simulink model "sim_plant"  (R2023a)
settings: configuration reference "config" (kept outside this file)
model workspace (MATLAB code in the model file):
  | cmdLim = Simulink.Parameter;
  | cmdLim.Value = 15;
  | cmdLim.Description = 'Limit for controlling the maximum surface command angle.';
  | cmdLim.Min = 0;
  | cmdLim.Max = 90;
  | cmdLim.DocUnits = 'deg';
  | 
  | dispGain = Simulink.Parameter;
  | dispGain.Value = 0.75;
  | dispGain.Description = 'Gain applied to the displacement error.';
  | dispGain.Min = 0;
  | dispGain.Max = [];
  | dispGain.DocUnits = 'deg/sec/deg';
  | 
  | dispLim = Simulink.Parameter;
  | dispLim.Value = 30;
  | dispLim.Description = 'Limit for controlling the maximum commanded angle.';
  | dispLim.Min = 0;
  | dispLim.Max = 180;
  | dispLim.DocUnits = 'deg';
  | 
  | intGain = Simulink.Parameter;
  | intGain.Value = 0.5;
  | intGain.Description = 'Gain applied to the integral error.';
  | intGain.Min = 0;
  | intGain.Max = [];
  | intGain.DocUnits = 'deg/sec/deg/sec';
  | 
  | intLim = Simulink.Parameter;
  | intLim.Value = 5;
  | intLim.Description = 'Limit for controlling the maximum commanded angle.';
  | intLim.Min = 0;
  | intLim.Max = 90;
  | intLim.DocUnits = 'deg';
  | 
  | rateGain = Simulink.Parameter;
  | rateGain.Value = 2;
  | rateGain.Description = 'Gain applied to the rate error.';
  | rateGain.Min = 0;
  | rateGain.Max = [];
  | rateGain.DocUnits = 'deg/deg/sec';
  | 
  | rateLim = Simulink.Parameter;
  | rateLim.Value = 6;
  | rateLim.Description = 'Limit for controlling the maximum commanded angle.';
  | rateLim.Min = 0;
  | rateLim.Max = 180;
  | rateLim.DocUnits = 'deg/sec';
  | 
  | hdgGain = Simulink.Parameter;
  | hdgGain.Value = 0.015;
libraries: eeTransforms x2, servo_hub_lib x1
settings Model: RequirementInfo={} %GIDa_fe9045fd_0412_4b6e_8206_617cc20e6fde  DataDictionary=model_config.sldd  Creator=Administrator  LastModifiedBy=Administrator
settings ConfigSetRef: SourceName=config

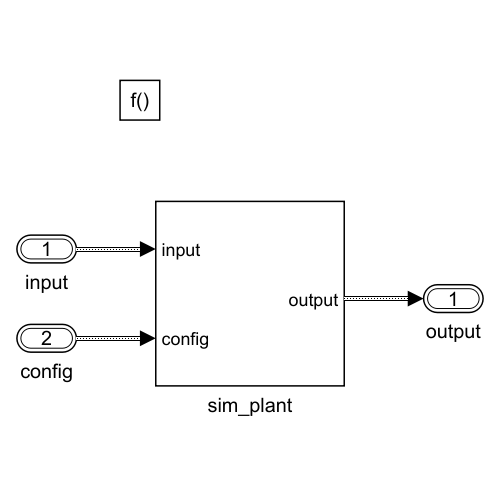
[thumbnail: Simulink's stored preview of the top-level diagram]
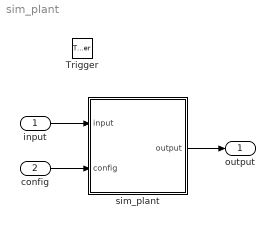
== system sim_plant ==
  input : Inport  OutDataTypeStr=Bus: SimPlantInput  BusOutputAsStruct=on
  config : Inport  Port=2  OutDataTypeStr=Bus: SimPlantConfig  BusOutputAsStruct=on
  Trigger : TriggerPort  TriggerType=function-call  VariantControl=(inherit)  PortDimensions=1
  sim_plant : Subsystem
  output : Outport  OutDataTypeStr=Bus: SimPlantOutput  BusOutputAsStruct=on
  wires:
  config/1 -> sim_plant/2(config)
  input/1 -> sim_plant/1(input)
  sim_plant/1(output) -> output/1

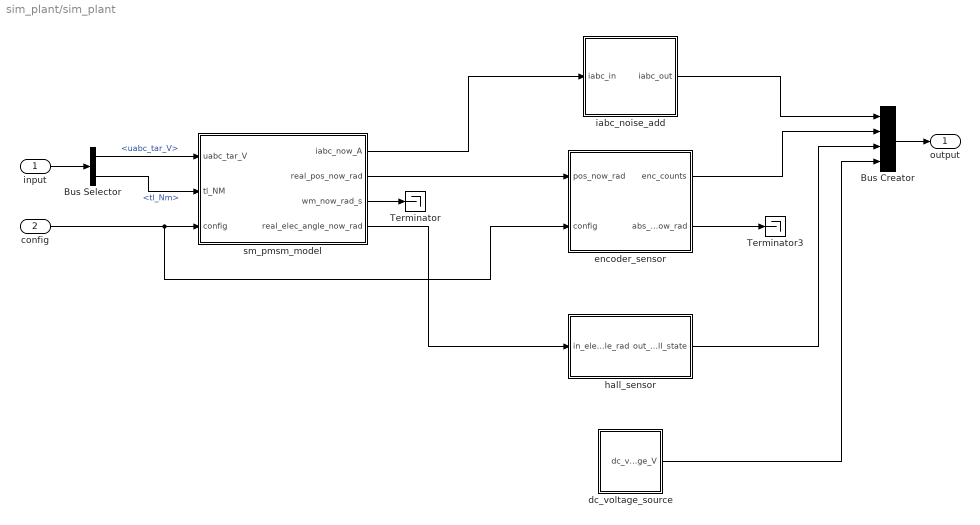
== system sim_plant/sim_plant ==
  input : Inport
  config : Inport  Port=2
  Bus Creator : BusCreator  Inputs=4  OutDataTypeStr=Bus: SimPlantOutput  NonVirtualBus=on
      settings: InheritFromInputs=off
  Bus Selector : BusSelector  OutputSignals=uabc_tar_V,tl_Nm
  Terminator : Terminator
  Terminator3 : Terminator
  dc_voltage_source : Subsystem
  encoder_sensor : Subsystem
  hall_sensor : Subsystem
  iabc_noise_add : Subsystem
  sm_pmsm_model : Subsystem
  output : Outport
  wires:
  sm_pmsm_model/2(real_pos_now_rad) -> encoder_sensor/1(pos_now_rad)
  Bus Selector/1 -> sm_pmsm_model/1(uabc_tar_V)  "<uabc_tar_V>"
  sm_pmsm_model/3(wm_now_rad_s) -> Terminator/1
  encoder_sensor/1(enc_counts) -> Bus Creator/2
  encoder_sensor/2(abs_pos_now_rad) -> Terminator3/1
  config/1 -> encoder_sensor/2(config), sm_pmsm_model/3(config)
  hall_sensor/1(out_hall_state) -> Bus Creator/3
  Bus Selector/2 -> sm_pmsm_model/2(tl_NM)  "<tl_Nm>"
  sm_pmsm_model/4(real_elec_angle_now_rad) -> hall_sensor/1(in_elec_angle_rad)
  Bus Creator/1 -> output/1
  input/1 -> Bus Selector/1
  sm_pmsm_model/1(iabc_now_A) -> iabc_noise_add/1(iabc_in)
  iabc_noise_add/1(iabc_out) -> Bus Creator/1
  dc_voltage_source/1(dc_voltage_V) -> Bus Creator/4

== system sim_plant/sim_plant/dc_voltage_source ==
  Add : Sum
  Data Type Conversion1 : DataTypeConversion  OutDataTypeStr=single  SaturateOnIntegerOverflow=off  RndMeth=Floor
  Uniform Random Number1 : UniformRandomNumber  Seed=4
  dc_bus_noise_V : Gain  Gain=0.1
  dc_voltage_base : Constant  Value=48  OutDataTypeStr=single  SampleTime=-1
  dc_voltage_V : Outport
  wires:
  dc_voltage_base/1 -> Add/1
  dc_bus_noise_V/1 -> Add/2  "noise"
  Uniform Random Number1/1 -> Data Type Conversion1/1
  Add/1 -> dc_voltage_V/1
  Data Type Conversion1/1 -> dc_bus_noise_V/1

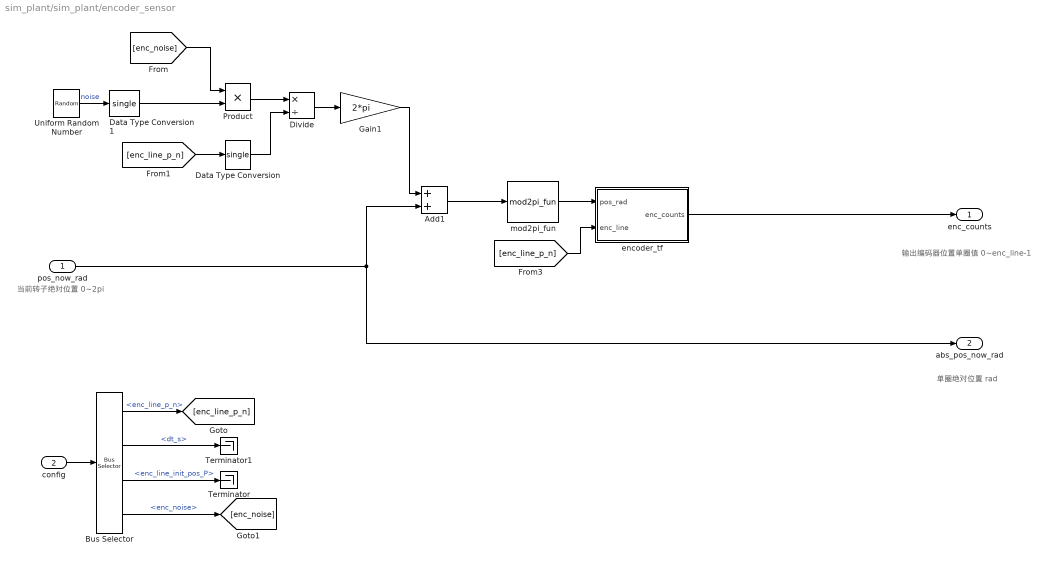
== system sim_plant/sim_plant/encoder_sensor ==
  note: 当前转子绝对位置 0~2pi
  note: 单圈绝对位置 rad
  note: 输出编码器位置单圈值 0~enc_line-1
  pos_now_rad : Inport
  config : Inport  Port=2
  Add1 : Sum
  Bus Selector : BusSelector  OutputSignals=enc_line_p_n,dt_s,enc_line_init_pos_P,enc_noise
  Data Type Conversion : DataTypeConversion  OutDataTypeStr=single  SaturateOnIntegerOverflow=off  RndMeth=Floor
  Data Type Conversion1 : DataTypeConversion  OutDataTypeStr=single  SaturateOnIntegerOverflow=off  RndMeth=Floor
  Divide : Product  Inputs=*/
  Gain1 : Gain  Gain=2*pi
  Product : Product
  Terminator : Terminator
  Terminator1 : Terminator
  Uniform Random Number : UniformRandomNumber
  encoder_tf : Subsystem
  mod2pi_fun : servo_hub_lib/fast_math/mod2pi_fun  SystemSampleTime=-1  VariantActivationTime=update diagram  Latency=0  AutoFrameSizeCalculation=off
      settings: LibrarySourceBlock=|
      | simulink/User-Defined
      | Functions/MATLAB Function
  enc_counts : Outport
  abs_pos_now_rad : Outport  Port=2
  wires:
  Data Type Conversion1/1 -> Product/2
  Uniform Random Number/1 -> Data Type Conversion1/1  "noise"
  encoder_tf/1(enc_counts) -> enc_counts/1
  Add1/1 -> mod2pi_fun/1
  mod2pi_fun/1 -> encoder_tf/1(pos_rad)
  pos_now_rad/1 -> Add1/2, abs_pos_now_rad/1
  Product/1 -> Divide/1
  [enc_line_p_n] -> Data Type Conversion/1
  Divide/1 -> Gain1/1
  config/1 -> Bus Selector/1
  Bus Selector/1 -> [enc_line_p_n]  "<enc_line_p_n>"
  Bus Selector/2 -> Terminator1/1  "<dt_s>"
  Bus Selector/3 -> Terminator/1  "<enc_line_init_pos_P>"
  Bus Selector/4 -> [enc_noise]  "<enc_noise>"
  [enc_noise] -> Product/1
  [enc_line_p_n] -> encoder_tf/2(enc_line)
  Data Type Conversion/1 -> Divide/2
  Gain1/1 -> Add1/1

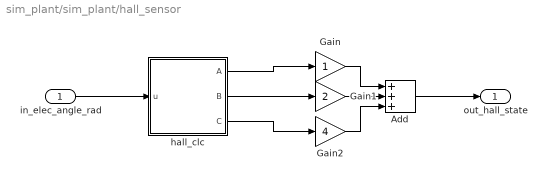
== system sim_plant/sim_plant/hall_sensor ==
  in_elec_angle_rad : Inport  OutDataTypeStr=single
  Add : Sum  Inputs=+++
  Gain : Gain  OutDataTypeStr=uint8
  Gain1 : Gain  Gain=2  OutDataTypeStr=uint8
  Gain2 : Gain  Gain=4  OutDataTypeStr=uint8
  hall_clc : MATLAB Function  TreatAsAtomicUnit=on
  out_hall_state : Outport  OutDataTypeStr=uint8
  wires:
  hall_clc/3(C) -> Gain2/1
  Add/1 -> out_hall_state/1
  hall_clc/1(A) -> Gain/1
  Gain1/1 -> Add/2
  Gain/1 -> Add/1
  in_elec_angle_rad/1 -> hall_clc/1(u)
  hall_clc/2(B) -> Gain1/1
  Gain2/1 -> Add/3

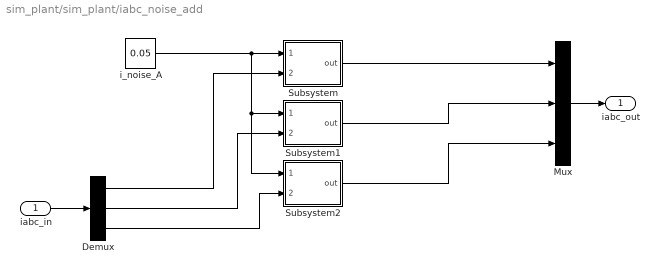
== system sim_plant/sim_plant/iabc_noise_add ==
  iabc_in : Inport
  Demux : Demux  Outputs=3
  Mux : Mux  Inputs=3
  Subsystem : Subsystem  TreatAsAtomicUnit=on
  Subsystem1 : Subsystem  TreatAsAtomicUnit=on
  Subsystem2 : Subsystem  TreatAsAtomicUnit=on
  i_noise_A : Constant  Value=0.05  OutDataTypeStr=single
  iabc_out : Outport
  wires:
  iabc_in/1 -> Demux/1
  Mux/1 -> iabc_out/1
  i_noise_A/1 -> Subsystem2/1(noise_amp), Subsystem1/1(noise_amp), Subsystem/1(noise_amp)
  Demux/1 -> Subsystem/2(source)
  Subsystem/1(out) -> Mux/1
  Subsystem1/1(out) -> Mux/2
  Subsystem2/1(out) -> Mux/3
  Demux/2 -> Subsystem1/2(source)
  Demux/3 -> Subsystem2/2(source)

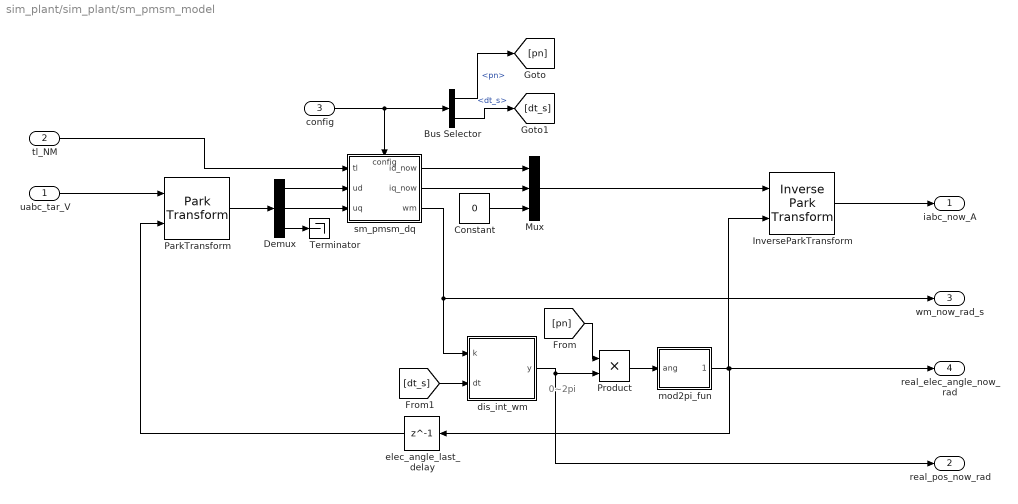
== system sim_plant/sim_plant/sm_pmsm_model ==
  note: 0~2pi
  uabc_tar_V : Inport  OutDataTypeStr=single  PortDimensions=3
  tl_NM : Inport  Port=2  OutDataTypeStr=single
  config : Inport  Port=3
  Bus Selector : BusSelector  OutputSignals=pn,dt_s
  Constant : Constant  Value=0  OutDataTypeStr=single  SampleTime=-1
  Demux : Demux  Outputs=3
  InverseParkTransform : eeTransforms/Inverse Park Transform  AxisAlignment=D-axis  PowerInvariant=off
      settings: LibrarySourceBlock=|
      | ee_sl_lib/Mathematical
      | Transforms/Inverse
      | Park Transform
  Mux : Mux  Inputs=3
  ParkTransform : eeTransforms/Park Transform  AxisAlignment=D-axis  PowerInvariant=off
      settings: LibrarySourceBlock=|
      | ee_sl_lib/Mathematical
      | Transforms/Park Transform
  Product : Product
  Terminator : Terminator
  dis_int_wm : Subsystem
  elec_angle_last_delay : Delay  DelayLength=1  StateName=elec_angle_last
  mod2pi_fun : MATLAB Function
  sm_pmsm_dq : Subsystem
      settings: PortSchema="{\"entries\":[{\"content\":{\"sides\":[{\"content\":{\"connectorIds\":[\"In1\",\"In2\",\"In3\"]},\"type\":\"ConnectorPlacement.EquallySpacedRectSide\",\"uuid\":\"d8cc84ce-9f3b-47a0-8bee-f47dde5345ac\"},{\"content\":{\"connectorIds\":[\"Out1\",\"Out2\",\"Out3\"],\"side\":\"RIGHT\"},\"type\":\"ConnectorPlacement.EquallySpacedRectSide\",\"uuid\":\"7a05c8dd-b607-4215-ae3a-55de450e01b9\"},{\"content\":{\"connectorIds\":[\"In4\"],\"side\":\"TOP\"},\"type\":\"ConnectorPlacement.EquallySpacedRectSide\",\"uuid\":\"29e5b71a-7e7a-40d5-8a8d-08d5a436dd58\"}]},\"type\":\"ConnectorPlacement.EquallySpacedConnector\",\"uuid\":\"95edc6c6-16f9-4a9f-9bec-fe8bb0215fcd\"}],\"packageUris\":[\"http://schema.mathworks.com/mf0/Connector/R2020b\"],\"version\":\"1.0\"}"
  iabc_now_A : Outport  OutDataTypeStr=single
  real_pos_now_rad : Outport  Port=2  OutDataTypeStr=single
  wm_now_rad_s : Outport  Port=3  OutDataTypeStr=single
  real_elec_angle_now_rad : Outport  Port=4  OutDataTypeStr=single
  wires:
  sm_pmsm_dq/2(iq_now) -> Mux/2
  InverseParkTransform/1 -> iabc_now_A/1
  Demux/3 -> Terminator/1
  sm_pmsm_dq/1(id_now) -> Mux/1
  sm_pmsm_dq/3(wm) -> dis_int_wm/1(k), wm_now_rad_s/1
  Constant/1 -> Mux/3
  Demux/2 -> sm_pmsm_dq/3(uq)
  Demux/1 -> sm_pmsm_dq/2(ud)
  dis_int_wm/1(y) -> real_pos_now_rad/1, Product/2
  tl_NM/1 -> sm_pmsm_dq/1(tl)
  ParkTransform/1 -> Demux/1
  Mux/1 -> InverseParkTransform/1
  uabc_tar_V/1 -> ParkTransform/1
  Product/1 -> mod2pi_fun/1(ang)
  mod2pi_fun/1(n_ang) -> InverseParkTransform/2, elec_angle_last_delay/1, real_elec_angle_now_rad/1
  elec_angle_last_delay/1 -> ParkTransform/2
  config/1 -> Bus Selector/1, sm_pmsm_dq/4(config)
  Bus Selector/1 -> [pn]  "<pn>"
  [pn] -> Product/1
  Bus Selector/2 -> [dt_s]  "<dt_s>"
  [dt_s] -> dis_int_wm/2(dt)

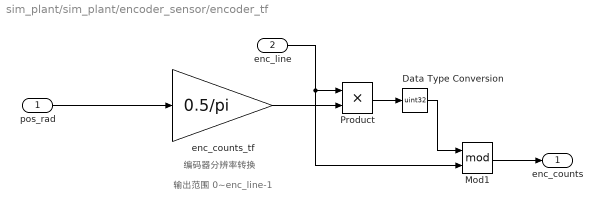
== system sim_plant/sim_plant/encoder_sensor/encoder_tf ==
  note: 输出范围 0~enc_line-1
  note: 编码器分辨率转换
  pos_rad : Inport  OutDataTypeStr=single
  enc_line : Inport  Port=2
  Data Type Conversion : DataTypeConversion  OutDataTypeStr=uint32  SaturateOnIntegerOverflow=off  RndMeth=Floor
  Mod1 : Math  Operator=mod
  Product : Product
  enc_counts_tf : Gain  Gain=0.5/pi
  enc_counts : Outport
  wires:
  enc_counts_tf/1 -> Product/2
  pos_rad/1 -> enc_counts_tf/1
  enc_line/1 -> Mod1/2, Product/1
  Mod1/1 -> enc_counts/1
  Product/1 -> Data Type Conversion/1
  Data Type Conversion/1 -> Mod1/1

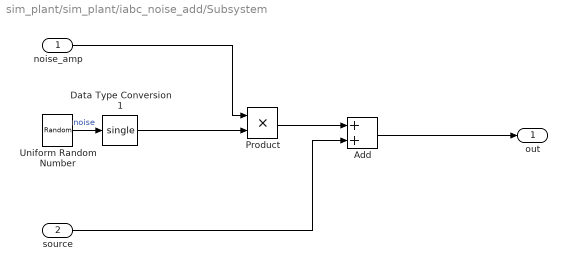
== system sim_plant/sim_plant/iabc_noise_add/Subsystem ==
  noise_amp : Inport
  source : Inport  Port=2
  Add : Sum
  Data Type Conversion1 : DataTypeConversion  OutDataTypeStr=single  SaturateOnIntegerOverflow=off  RndMeth=Floor
  Product : Product
  Uniform Random Number : UniformRandomNumber  Seed=1
  out : Outport
  wires:
  Product/1 -> Add/1
  Uniform Random Number/1 -> Data Type Conversion1/1  "noise"
  Data Type Conversion1/1 -> Product/2
  noise_amp/1 -> Product/1
  Add/1 -> out/1
  source/1 -> Add/2

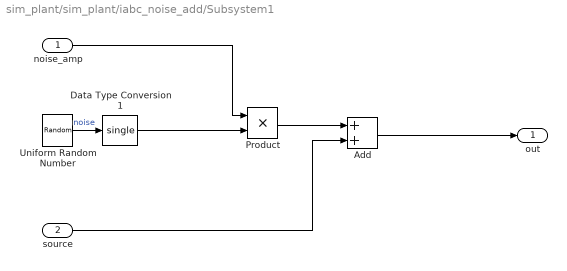
== system sim_plant/sim_plant/iabc_noise_add/Subsystem1 ==
  noise_amp : Inport
  source : Inport  Port=2
  Add : Sum
  Data Type Conversion1 : DataTypeConversion  OutDataTypeStr=single  SaturateOnIntegerOverflow=off  RndMeth=Floor
  Product : Product
  Uniform Random Number : UniformRandomNumber  Seed=2
  out : Outport
  wires:
  Product/1 -> Add/1
  Uniform Random Number/1 -> Data Type Conversion1/1  "noise"
  Data Type Conversion1/1 -> Product/2
  noise_amp/1 -> Product/1
  Add/1 -> out/1
  source/1 -> Add/2

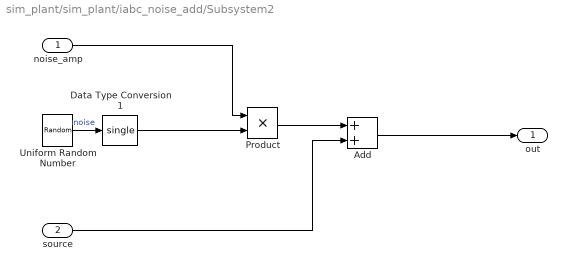
== system sim_plant/sim_plant/iabc_noise_add/Subsystem2 ==
  noise_amp : Inport
  source : Inport  Port=2
  Add : Sum
  Data Type Conversion1 : DataTypeConversion  OutDataTypeStr=single  SaturateOnIntegerOverflow=off  RndMeth=Floor
  Product : Product
  Uniform Random Number : UniformRandomNumber  Seed=3
  out : Outport
  wires:
  Product/1 -> Add/1
  Uniform Random Number/1 -> Data Type Conversion1/1  "noise"
  Data Type Conversion1/1 -> Product/2
  noise_amp/1 -> Product/1
  Add/1 -> out/1
  source/1 -> Add/2

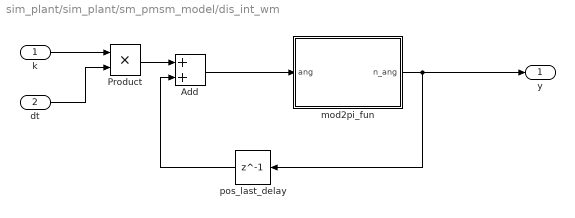
== system sim_plant/sim_plant/sm_pmsm_model/dis_int_wm ==
  k : Inport  OutDataTypeStr=single
  dt : Inport  Port=2
  Add : Sum
  Product : Product
  mod2pi_fun : MATLAB Function
  pos_last_delay : Delay  DelayLength=1  StateName=pos_last
  y : Outport  OutDataTypeStr=single
  wires:
  k/1 -> Product/1
  Product/1 -> Add/1
  mod2pi_fun/1(n_ang) -> y/1, pos_last_delay/1
  Add/1 -> mod2pi_fun/1(ang)
  pos_last_delay/1 -> Add/2
  dt/1 -> Product/2

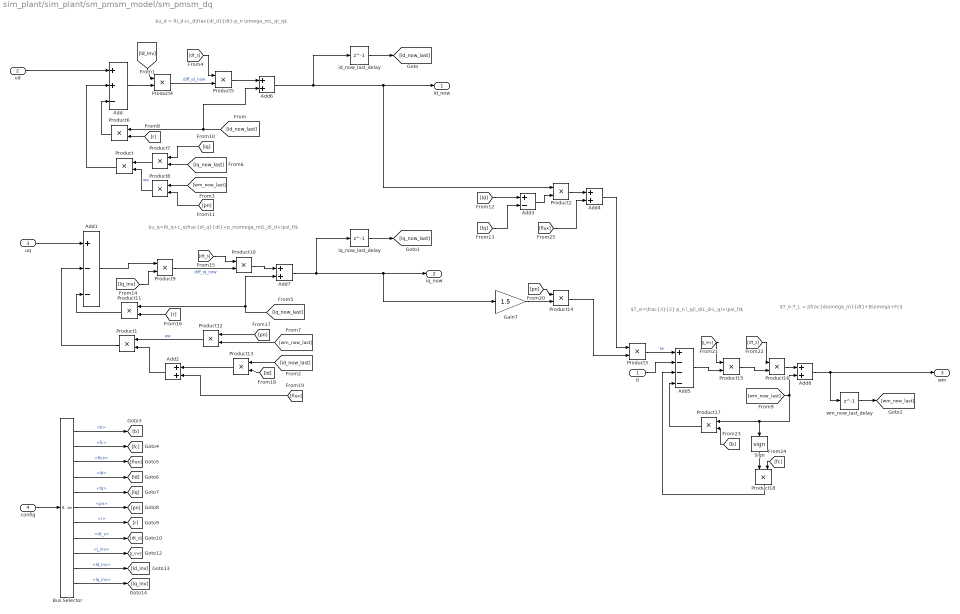
== system sim_plant/sim_plant/sm_pmsm_model/sm_pmsm_dq ==
  note: $u_d = Ri_d+L_d\frac{di_d}{dt}-p_n \omega_mL_qi_q$
  note: $u_q=Ri_q+L_q\frac{di_q}{dt}+p_n\omega_m(L_di_d+\psi_f)$
  note: $T_e=\frac{3}{2} p_n i_q(i_d(L_d-L_q)+\psi_f)$
  note: $T_e-T_L = J\frac{d\omega_m}{dt}+B\omega+Fc$
  tl : Inport
  ud : Inport  Port=2
  uq : Inport  Port=3
  config : Inport  Port=4
  Add : Sum  Inputs=++-
  Add1 : Sum  Inputs=+--
  Add{2,4,6..8} (5 alike) : Sum
  Add3 : Sum  Inputs=+-
  Add5 : Sum  Inputs=+---
  Bus Selector : BusSelector  OutputSignals=b,fc,flux,ld,lq,pn,r,dt_s,j_inv,ld_inv,lq_inv
  Gain7 : Gain  Gain=1.5
  Product{,1..18} (19 alike) : Product
  Sign : Signum
  id_now_last_delay : Delay  DelayLength=1  StateName=id_now_last
  iq_now_last_delay : Delay  DelayLength=1  StateName=iq_now_last
  wm_now_last_delay : Delay  DelayLength=1  StateName=wm_now_last
  id_now : Outport
  iq_now : Outport  Port=2
  wm : Outport  Port=3
  wires:
  Add6/1 -> Product2/1, id_now/1, id_now_last_delay/1
  Product7/1 -> Product/1
  Product2/1 -> Add4/1
  Sign/1 -> Product18/1
  [flux] -> Add4/2
  Product/1 -> Add/2
  Product6/1 -> Add/3
  Gain7/1 -> Product14/2
  Product13/1 -> Add2/1
  Product3/1 -> Add5/1  "te"
  Product11/1 -> Add1/3
  ud/1 -> Add/1
  [lq] -> Add3/2
  Product18/1 -> Add5/3
  Add1/1 -> Product9/1
  Product17/1 -> Add5/4
  [ld] -> Add3/1
  Product1/1 -> Add1/2
  tl/1 -> Add5/2
  Add3/1 -> Product2/2
  Add7/1 -> iq_now_last_delay/1, Gain7/1, iq_now/1
  Add2/1 -> Product1/2
  Add/1 -> Product4/2
  Add5/1 -> Product15/2
  Add8/1 -> wm/1, wm_now_last_delay/1
  id_now_last_delay/1 -> [id_now_last]
  iq_now_last_delay/1 -> [iq_now_last]
  [id_now_last] -> Product13/1
  wm_now_last_delay/1 -> [wm_now_last]
  [wm_now_last] -> Product8/1
  [wm_now_last] -> Product17/1, Sign/1, Add8/2
  [iq_now_last] -> Product7/2
  [id_now_last] -> Product6/1, Add6/2
  Product4/1 -> Product5/2  "diff_id_now"
  Product5/1 -> Add6/1
  uq/1 -> Add1/1
  Product8/1 -> Product/2  "we"
  Product12/1 -> Product1/1  "we"
  [wm_now_last] -> Product12/2
  [flux] -> Add2/2
  [iq_now_last] -> Add7/2, Product11/1
  Product10/1 -> Add7/1
  Product9/1 -> Product10/2  "diff_iq_now"
  Product16/1 -> Add8/1
  Product15/1 -> Product16/2
  Add4/1 -> Product3/1
  Product14/1 -> Product3/2
  config/1 -> Bus Selector/1
  Bus Selector/1 -> [b]  "<b>"
  Bus Selector/2 -> [fc]  "<fc>"
  Bus Selector/3 -> [flux]  "<flux>"
  Bus Selector/4 -> [ld]  "<ld>"
  Bus Selector/5 -> [lq]  "<lq>"
  Bus Selector/6 -> [pn]  "<pn>"
  Bus Selector/7 -> [r]  "<r>"
  Bus Selector/8 -> [dt_s]  "<dt_s>"
  Bus Selector/9 -> [j_inv]  "<j_inv>"
  Bus Selector/10 -> [ld_inv]  "<ld_inv>"
  Bus Selector/11 -> [lq_inv]  "<lq_inv>"
  [ld_inv] -> Product4/1
  [dt_s] -> Product5/1
  [r] -> Product6/2
  [lq] -> Product7/1
  [pn] -> Product8/2
  [lq_inv] -> Product9/2
  [dt_s] -> Product10/1
  [r] -> Product11/2
  [pn] -> Product12/1
  [ld] -> Product13/2
  [pn] -> Product14/1
  [j_inv] -> Product15/1
  [dt_s] -> Product16/1
  [b] -> Product17/2
  [fc] -> Product18/2

== matlab function sim_plant/sm_pmsm_model/dis_int_wm/mod2pi_fun ==
  data: ang input; n_ang output
function n_ang = mod2pi(ang)
    % 将角度限制在0到2π范围内
    TWO_PI = single(2*pi);
    n_ang = single(ang);
    while n_ang < 0
        n_ang = n_ang + TWO_PI;
    end
    while n_ang >= TWO_PI
        n_ang = n_ang - TWO_PI;
    end
end

== matlab function sim_plant/sm_pmsm_model/mod2pi_fun ==
  data: ang input; n_ang output
function n_ang = mod2pi(ang)
    % 将角度限制在0到2π范围内
    TWO_PI = single(2*pi);
    n_ang = single(ang);
    while n_ang < 0
        n_ang = n_ang + TWO_PI;
    end
    while n_ang >= TWO_PI
        n_ang = n_ang - TWO_PI;
    end
end

== matlab function sim_plant/hall_sensor/hall_clc ==
  data: u input; A output; B output; C output
function [A,B,C] = HALL_Sensro(u)
sita = u*360/(2*pi);

if (sita>=0 && sita<30) || (sita>=330 && sita<=360)
    A = 1;
    B = 1;
    C = 0;
elseif sita>=30 && sita<90
    A = 0;
    B = 1;
    C = 0;
elseif sita >=90 && sita <150
    A = 0;
    B = 1;
    C = 1;
elseif sita >=150 && sita <210
    A = 0;
    B = 0;
    C = 1;
elseif sita >=210 && sita <270
    A = 1;
    B = 0;
    C = 1;
elseif sita >=270 && sita <330
    A = 1;
    B = 0;
    C = 0;
else 
    A = 0;
    B = 0;
    C = 0;
end
